simulink model "u14042021"  (R2014b)
settings: Solver=ode45  StartTime=0.0  StopTime=12.8  RelTol=1e-3
values from neighbouring files (symbols this model uses):
  Td = []    [Sint_Bode (4).m]    (also in Sint_Bode.m)
  Tn = []    [Sint_Bode (4).m]    (also in Sint_Bode.m)
settings Model: Creator=maksimka  LastModifiedBy=maksimka

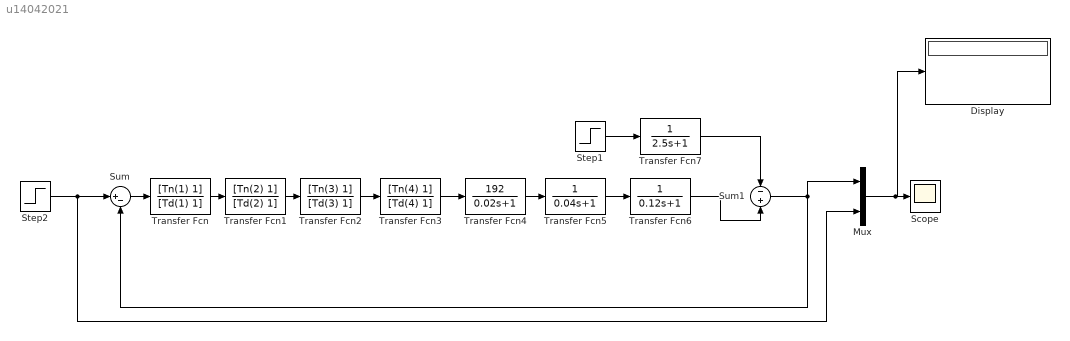
== system u14042021 ==
  Display : Display
  Mux : Mux  Inputs=2
  Scope : Scope
  Step1 : Step  Time=6.4  After=0.5  SampleTime=0
  Step2 : Step  Time=0  SampleTime=0
  Sum : Sum  Inputs=|+-
  Sum1 : Sum  Inputs=-+
  Transfer Fcn : TransferFcn  Numerator=[Tn(1) 1]  Denominator=[Td(1) 1]
  Transfer Fcn1 : TransferFcn  Numerator=[Tn(2) 1]  Denominator=[Td(2) 1]
  Transfer Fcn2 : TransferFcn  Numerator=[Tn(3) 1]  Denominator=[Td(3) 1]
  Transfer Fcn3 : TransferFcn  Numerator=[Tn(4) 1]  Denominator=[Td(4) 1]
  Transfer Fcn4 : TransferFcn  Numerator=[192]  Denominator=[0.02 1]
  Transfer Fcn5 : TransferFcn  Denominator=[0.04 1]
  Transfer Fcn6 : TransferFcn  Denominator=[0.12 1]
  Transfer Fcn7 : TransferFcn  Denominator=[2.5 1]
  wires:
  Step2/1 -> Mux/2, Sum/1
  Transfer Fcn/1 -> Transfer Fcn1/1
  Transfer Fcn1/1 -> Transfer Fcn2/1
  Transfer Fcn2/1 -> Transfer Fcn3/1
  Transfer Fcn4/1 -> Transfer Fcn5/1
  Transfer Fcn5/1 -> Transfer Fcn6/1
  Sum/1 -> Transfer Fcn/1
  Transfer Fcn6/1 -> Sum1/2
  Sum1/1 -> Mux/1, Sum/2
  Step1/1 -> Transfer Fcn7/1
  Mux/1 -> Display/1, Scope/1
  Transfer Fcn7/1 -> Sum1/1
  Transfer Fcn3/1 -> Transfer Fcn4/1
